simulink model "sampleModel1448_1_sub_sub_sub"  (R2023a)
settings: Solver=VariableStepAuto  StartTime=0.0  StopTime=10.0  RelTol=1e-3
libraries: hdlsllib x6, simulink x1
settings Model: Creator=user1  LastModifiedBy=user1

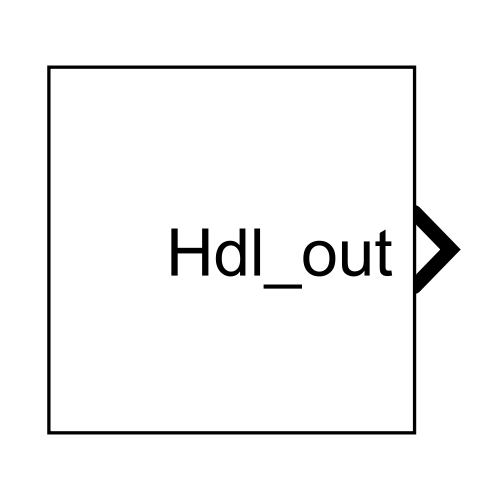
[thumbnail: Simulink's stored preview of the top-level diagram]
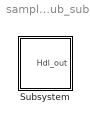
== system sampleModel1448_1_sub_sub_sub ==
  Subsystem : Subsystem

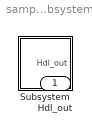
== system sampleModel1448_1_sub_sub_sub/Subsystem ==
  Subsystem : Subsystem
  Hdl_out : Outport  OutDataTypeStr=uint8

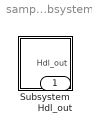
== system sampleModel1448_1_sub_sub_sub/Subsystem/Subsystem ==
  Subsystem : Subsystem
  Hdl_out : Outport  OutDataTypeStr=uint8

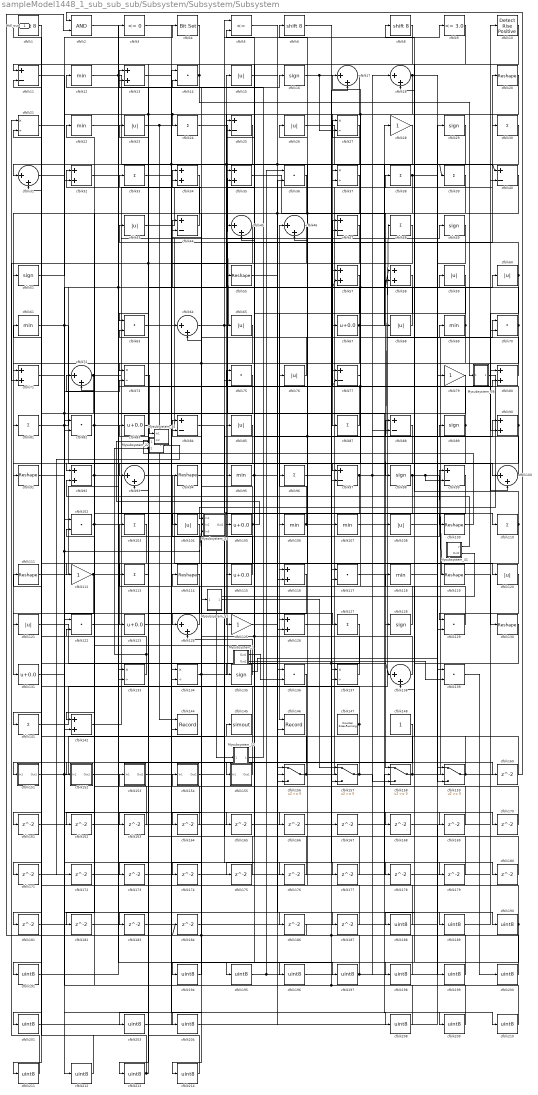
== system sampleModel1448_1_sub_sub_sub/Subsystem/Subsystem/Subsystem ==
  Mysubsystem_1 : Subsystem  TreatAsAtomicUnit=on  RTWFcnName=Mysubsystem_1
      settings: RTWFcnNameOpts=User specified  RTWFileNameOpts=Use function name
  Mysubsystem_12 : Subsystem  TreatAsAtomicUnit=on  RTWFcnName=Mysubsystem_12
      settings: RTWFcnNameOpts=User specified  RTWFileNameOpts=Use function name
  Mysubsystem_22 : Subsystem  TreatAsAtomicUnit=on  RTWFcnName=Mysubsystem_22
      settings: RTWFcnNameOpts=User specified  RTWFileNameOpts=Use function name
  Mysubsystem_23 : Subsystem  TreatAsAtomicUnit=on  RTWFcnName=Mysubsystem_23
      settings: RTWFcnNameOpts=User specified  RTWFileNameOpts=Use function name
  Mysubsystem_34 : Subsystem  TreatAsAtomicUnit=on  RTWFcnName=Mysubsystem_34
      settings: RTWFcnNameOpts=User specified  RTWFileNameOpts=Use function name
  Mysubsystem_36 : Subsystem  TreatAsAtomicUnit=on  RTWFcnName=Mysubsystem_36
      settings: RTWFcnNameOpts=User specified  RTWFileNameOpts=Use function name
  Mysubsystem_41 : Subsystem  TreatAsAtomicUnit=on  RTWFcnName=Mysubsystem_41
      settings: RTWFcnNameOpts=User specified  RTWFileNameOpts=Use function name
  Mysubsystem_51 : Subsystem  TreatAsAtomicUnit=on  RTWFcnName=Mysubsystem_51
      settings: RTWFcnNameOpts=User specified  RTWFileNameOpts=Use function name
  cfblk1 : ArithShift  BitShiftNumber=8
  cfblk10 : hdlsllib/Logic and Bit Operations/Detect Rise Positive  vinit=0  OutDataTypeStr=uint8
  cfblk{17..18,31,45..46,64,72,93,100,124,138} (11 alike) : Sum  Inputs=|++  OutDataTypeStr=uint8
  cfblk{14,36,63,70,75,82,102,117,122,129,136,139} (12 alike) : DotProduct  OutDataTypeStr=uint8
  cfblk{24,30,33,38..39,48,81,87,96,103,110,113,127,141} (14 alike) : Sum  Inputs=+  OutDataTypeStr=uint8
  cfblk{15,23,26,43,59..60,65,68,76,85,104,108,120..121} (14 alike) : Abs  OutDataTypeStr=uint8  SaturateOnIntegerOverflow=off
  cfblk{67,83,105,115,123,131} (6 alike) : Bias  Bias=0.0  SaturateOnIntegerOverflow=off
  cfblk{12,22,61,69,95,106..107,118} (8 alike) : MinMax  OutDataTypeStr=uint8
  cfblk{20,55,91,94,109,111,114,119,130} (9 alike) : Reshape
  cfblk{11,25,40,44,47,77,84,88,97,99} (10 alike) : Sum  Inputs=+-  OutDataTypeStr=uint8
  cfblk{28,79,112,125} (4 alike) : Gain  OutDataTypeStr=uint8
  cfblk{13,32,34..35,57..58,71,80,90,92,116,126,142} (13 alike) : Sum  OutDataTypeStr=uint8
  cfblk{16,29,49,51,89,98,128,135} (8 alike) : Signum
  cfblk{21,27,37,73,133..134,137} (7 alike) : Product  Inputs=*/  OutDataTypeStr=uint8  RndMeth=Zero  SaturateOnIntegerOverflow=on
  cfblk144 : Record  FileSettingsInternal="{\"entries\":[{\"content\":{\"excelSettings\":{\"content\":{},\"type\":\"Streamout.ExcelSettings\"}},\"type\":\"Streamout.FileSettingStorage\",\"uuid\":\"\"}],\"packageUris\":[\"http:\\/\\/schema.mathworks.com\\/mf0\\/streamout_blocks\\/R2020a\"],\"version\":\"1.0\"}"  Layout=[1 1]  SignalsInternal="{\"entries\":[{\"content\":{\"signals\":[{\"content\":{\"blockPath\":[],\"dimensions\":[1],\"domain\":\"\",\"lineColor\":\"#a2142f\",\"plots\":[1],\"port\":1,\"signalID\":16776,\"signalName\":\"cfblk23\"},\"type\":\"RecordBlkView.Signal\",\"uuid\":\"\"},{\"content\":{\"blockPath\":[],\"dimensions\":[1],\"domain\":\"\",\"lineColor\":\"#139fff\",\"plots\":[1],\"port\":2,\"signalID\":16779,\"signalName\":\"cfblk97\"},\"type\":\"RecordBlkView.Signal\",\"uuid\":\"\"}]},\"type\":\"RecordBlkView.InputSignals\",\"uuid\":\"\"}],\"packageUris\":[\"http:\\/\\/schema.mathworks.com\\/mf0\\/streamout_blocks\\/R2020a\"],\"version\":\"1.0\"}"  VisualizationBindings="{\"xyplotplugin\":{\"info\":[{\"series\":[{\"bindingParametersList\":[{\"parameter\":\"X-Axis\",\"signalID\":16776,\"signalName\":\"cfblk23\"},{\"parameter\":\"Y-Axis\",\"signalID\":16779,\"signalName\":\"cfblk97\"}],\"seriesID\":34221}],\"subplotID\":1}]}}"  CompatibilityTag=XY  st=-1
  cfblk145 : ToWorkspace  VariableName=simout  SaveFormat=Timeseries  SampleTime=-1
  cfblk146 : Record  FileSettingsInternal="{\"entries\":[{\"content\":{\"excelSettings\":{\"content\":{},\"type\":\"Streamout.ExcelSettings\"}},\"type\":\"Streamout.FileSettingStorage\",\"uuid\":\"\"}],\"packageUris\":[\"http:\\/\\/schema.mathworks.com\\/mf0\\/streamout_blocks\\/R2020a\"],\"version\":\"1.0\"}"  Layout=[1 1]  SignalsInternal="{\"entries\":[{\"content\":{\"signals\":[{\"content\":{\"blockPath\":[],\"dimensions\":[1],\"domain\":\"\",\"lineColor\":\"#a2142f\",\"plots\":[1],\"port\":1,\"signalID\":16784,\"signalName\":\"cfblk57\"},\"type\":\"RecordBlkView.Signal\",\"uuid\":\"\"},{\"content\":{\"blockPath\":[],\"dimensions\":[1],\"domain\":\"\",\"lineColor\":\"#139fff\",\"plots\":[1],\"port\":2,\"signalID\":16787,\"signalName\":\"cfblk29\"},\"type\":\"RecordBlkView.Signal\",\"uuid\":\"\"}]},\"type\":\"RecordBlkView.InputSignals\",\"uuid\":\"\"}],\"packageUris\":[\"http:\\/\\/schema.mathworks.com\\/mf0\\/streamout_blocks\\/R2020a\"],\"version\":\"1.0\"}"  VisualizationBindings="{\"xyplotplugin\":{\"info\":[{\"series\":[{\"bindingParametersList\":[{\"parameter\":\"X-Axis\",\"signalID\":16784,\"signalName\":\"cfblk57\"},{\"parameter\":\"Y-Axis\",\"signalID\":16787,\"signalName\":\"cfblk29\"}],\"seriesID\":57294}],\"subplotID\":1}]}}"  CompatibilityTag=XY  st=-1
  cfblk147 : hdlsllib/Sources/Counter Free-Running  NumBits=16  tsamp=-1
  cfblk148 : Constant  OutDataTypeStr=uint8  SampleTime=-1
  cfblk151 : Subsystem
      settings: LibrarySourceBlock=|
      | hdlsllib/Ports &
      | Subsystems/Subsystem
  cfblk152 : Subsystem
      settings: LibrarySourceBlock=|
      | hdlsllib/Ports &
      | Subsystems/Subsystem
  cfblk153 : Subsystem
      settings: LibrarySourceBlock=|
      | hdlsllib/Ports &
      | Subsystems/Subsystem
  cfblk154 : Subsystem
      settings: LibrarySourceBlock=|
      | hdlsllib/Ports &
      | Subsystems/Subsystem
  cfblk155 : Subsystem
      settings: LibrarySourceBlock=|
      | hdlsllib/Ports &
      | Subsystems/Subsystem
  cfblk{156..159} (4 alike) : Switch  OutDataTypeStr=uint8  SaturateOnIntegerOverflow=off  InputSameDT=off
  cfblk{160..184,186..187} (27 alike) : Delay  SampleTime=1
  cfblk{188..191,194..201,203..204,208..214} (21 alike) : DataTypeConversion  OutDataTypeStr=uint8  SaturateOnIntegerOverflow=off  RndMeth=Floor
  cfblk2 : Logic  AllPortsSameDT=off  OutDataTypeStr=boolean
  cfblk3 : hdlsllib/Logic and Bit Operations/Compare To Zero  relop=<=  OutDataTypeStr=uint8
  cfblk4 : simulink/Logic and Bit Operations/Bit Set  iBit=0
      settings: LibrarySourceBlock=|
      | hdlsllib/Logic and Bit
      | Operations/Bit Set
  cfblk5 : RelationalOperator  Operator=<=  OutDataTypeStr=boolean  InputSameDT=off
  cfblk6 : ArithShift  BitShiftNumber=8
  cfblk8 : ArithShift  BitShiftNumber=8
  cfblk9 : hdlsllib/Logic and Bit Operations/Compare To Constant  relop=<=  const=3.0  OutDataTypeStr=uint8
  Hdl_out : Outport  OutDataTypeStr=uint8
  wires:
  cfblk142/1 -> cfblk49/1
  cfblk157/1 -> cfblk158/3, cfblk155/1(In1)
  cfblk134/1 -> cfblk20/1, Mysubsystem_51/1(In1)
  cfblk156/1 -> cfblk145/1, cfblk38/1
  cfblk3/1 -> cfblk190/1
  cfblk106/1 -> cfblk109/1, cfblk46/1
  cfblk34/1 -> cfblk131/1
  cfblk93/1 -> cfblk120/1
  cfblk92/1 -> cfblk112/1, cfblk110/1
  cfblk17/1 -> cfblk87/1
  cfblk89/1 -> cfblk161/1, cfblk35/1
  cfblk25/1 -> cfblk84/2, cfblk125/1
  cfblk14/1 -> cfblk11/1, Mysubsystem_36/1(In1)
  cfblk57/1 -> cfblk146/1
  cfblk46/1 -> cfblk81/1
  cfblk5/1 -> cfblk160/1, cfblk39/1
  cfblk110/1 -> cfblk174/1, cfblk58/2
  cfblk8/1 -> cfblk93/1
  cfblk88/1 -> cfblk92/1
  cfblk85/1 -> cfblk91/1
  cfblk4/1 -> cfblk133/2
  cfblk100/1 -> cfblk45/2, cfblk6/1
  cfblk83/1 -> cfblk47/1
  cfblk108/1 -> cfblk29/1
  cfblk147/1 -> cfblk211/1, cfblk44/2
  cfblk67/1 -> cfblk181/1, cfblk44/1, cfblk28/1
  cfblk48/1 -> cfblk116/1
  cfblk90/1 -> cfblk204/1, cfblk47/2
  cfblk99/1 -> cfblk116/2
  cfblk115/1 -> cfblk94/1
  cfblk129/1 -> cfblk114/1
  cfblk141/1 -> cfblk60/1
  cfblk103/1 -> cfblk123/1
  cfblk76/1 -> cfblk12/1
  cfblk28/1 -> cfblk31/1
  cfblk82/1 -> cfblk182/1, cfblk58/1, cfblk16/1
  cfblk111/1 -> cfblk80/2
  cfblk158/1 -> cfblk31/2, cfblk70/1
  cfblk112/1 -> cfblk99/1, cfblk151/1(In1)
  cfblk87/1 -> cfblk13/1
  cfblk18/1 -> cfblk100/1, cfblk97/1, cfblk24/1, cfblk183/1, cfblk32/2
  cfblk51/1 -> cfblk4/1
  cfblk70/1 -> cfblk138/2, cfblk8/1
  cfblk138/1 -> cfblk96/1
  cfblk105/1 -> cfblk84/1, cfblk124/1
  cfblk13/1 -> cfblk64/1
  cfblk59/1 -> cfblk158/1
  cfblk122/1 -> cfblk197/1
  cfblk151/1(Out1) -> cfblk176/1, cfblk75/2
  cfblk35/1 -> cfblk128/1
  cfblk36/1 -> cfblk121/1
  cfblk29/1 -> cfblk65/1, cfblk146/2
  cfblk97/1 -> cfblk144/2, cfblk88/2, cfblk48/1
  cfblk38/1 -> cfblk71/1, cfblk159/1
  cfblk61/1 -> cfblk186/1, cfblk115/1
  cfblk128/1 -> cfblk27/1, cfblk77/2
  cfblk12/1 -> cfblk100/2, cfblk67/1
  cfblk77/1 -> cfblk57/2, cfblk17/1
  cfblk68/1 -> cfblk23/1
  cfblk137/1 -> cfblk45/1, cfblk34/1
  cfblk123/1 -> cfblk127/1
  cfblk81/1 -> cfblk73/2, cfblk15/1
  cfblk6/1 -> cfblk169/1, cfblk138/1
  cfblk21/1 -> cfblk210/1
  cfblk33/1 -> cfblk208/1
  cfblk102/1 -> cfblk168/1, cfblk22/1
  cfblk9/1 -> cfblk135/1
  cfblk139/1 -> cfblk200/1
  cfblk2/1 -> cfblk157/2
  cfblk133/1 -> cfblk111/1, Mysubsystem_22/2(In2)
  cfblk72/1 -> cfblk142/2, cfblk30/1
  cfblk39/1 -> cfblk106/1, cfblk194/1, cfblk126/2
  cfblk120/1 -> cfblk129/1
  cfblk98/1 -> cfblk99/2, cfblk119/1, cfblk152/1(In1), cfblk105/1
  cfblk117/1 -> cfblk69/1
  cfblk44/1 -> cfblk32/1
  cfblk159/1 -> cfblk118/1, cfblk2/1
  cfblk124/1 -> cfblk103/1
  cfblk20/1 -> cfblk95/1
  cfblk148/1 -> cfblk157/3
  cfblk121/1 -> cfblk156/2
  cfblk94/1 -> cfblk98/1
  cfblk95/1 -> cfblk35/2, cfblk89/1
  cfblk32/1 -> cfblk85/1
  cfblk64/1 -> cfblk9/1, cfblk108/1
  cfblk119/1 -> cfblk130/1
  cfblk118/1 -> cfblk90/1
  cfblk135/1 -> cfblk124/2
  cfblk60/1 -> cfblk43/1, cfblk90/2
  cfblk27/1 -> cfblk76/1
  cfblk113/1 -> cfblk213/1
  cfblk37/1 -> cfblk137/2
  cfblk114/1 -> cfblk134/2
  cfblk155/1(Out1) -> cfblk61/1
  cfblk24/1 -> cfblk107/1
  cfblk43/1 -> cfblk25/1
  cfblk69/1 -> cfblk18/2, cfblk164/1, cfblk163/1
  cfblk23/1 -> cfblk144/1, cfblk55/1, cfblk40/1
  cfblk30/1 -> cfblk63/1
  cfblk49/1 -> cfblk159/2
  cfblk131/1 -> cfblk59/1
  cfblk152/1(Out1) -> cfblk75/1
  cfblk1/1 -> cfblk51/1
  cfblk47/1 -> cfblk71/2, cfblk73/1
  cfblk80/1 -> cfblk5/2
  cfblk75/1 -> cfblk82/2, cfblk141/1
  cfblk40/1 -> cfblk72/2
  cfblk79/1 -> cfblk195/1
  cfblk154/1(Out1) -> cfblk88/1
  cfblk11/1 -> cfblk126/1
  cfblk22/1 -> cfblk104/1
  cfblk26/1 -> cfblk68/1
  cfblk16/1 -> cfblk179/1, cfblk27/2
  cfblk160/1 -> cfblk133/1
  cfblk161/1 -> cfblk156/1
  cfblk65/1 -> cfblk162/1
  cfblk162/1 -> cfblk37/2
  cfblk163/1 -> cfblk72/1
  cfblk164/1 -> cfblk63/2
  cfblk71/1 -> cfblk165/1
  cfblk165/1 -> cfblk77/1
  cfblk153/1(Out1) -> cfblk166/1
  cfblk166/1 -> cfblk46/2
  cfblk126/1 -> cfblk167/1
  cfblk167/1 -> cfblk40/2
  cfblk169/1 -> cfblk13/2
  cfblk96/1 -> cfblk170/1
  cfblk170/1 -> cfblk34/2
  cfblk45/1 -> cfblk171/1
  cfblk171/1 -> cfblk137/1
  cfblk172/1 -> cfblk117/2
  cfblk116/1 -> cfblk173/1
  cfblk173/1 -> cfblk158/2
  cfblk174/1 -> cfblk80/1
  cfblk58/1 -> cfblk175/1
  cfblk175/1 -> cfblk5/1
  cfblk176/1 -> cfblk64/2
  cfblk125/1 -> cfblk177/1
  cfblk177/1 -> cfblk25/2
  cfblk84/1 -> cfblk178/1
  cfblk178/1 -> cfblk70/2
  cfblk179/1 -> cfblk93/2
  cfblk31/1 -> cfblk180/1
  cfblk180/1 -> cfblk134/1
  cfblk181/1 -> cfblk129/2
  cfblk182/1 -> cfblk156/3
  cfblk183/1 -> cfblk36/2
  cfblk184/1 -> cfblk17/2
  cfblk186/1 -> cfblk2/2
  cfblk55/1 -> cfblk187/1
  cfblk187/1 -> cfblk1/1
  cfblk10/1 -> cfblk188/1
  cfblk188/1 -> cfblk26/1
  cfblk15/1 -> cfblk189/1
  cfblk189/1 -> cfblk10/1
  cfblk190/1 -> cfblk214/1, cfblk83/1
  cfblk104/1 -> cfblk191/1
  cfblk191/1 -> cfblk3/1
  cfblk195/1 -> cfblk36/1, cfblk97/2
  cfblk63/1 -> cfblk196/1
  cfblk196/1 -> cfblk79/1
  cfblk197/1 -> cfblk18/1, cfblk37/1, cfblk82/1
  cfblk130/1 -> cfblk198/1
  cfblk198/1 -> cfblk122/1
  cfblk168/1 -> cfblk199/1
  cfblk199/1 -> cfblk122/2
  cfblk200/1 -> cfblk117/1, cfblk154/1(In1), cfblk184/1
  cfblk127/1 -> cfblk201/1
  cfblk201/1 -> cfblk139/1
  cfblk136/1 -> cfblk203/1
  cfblk203/1 -> cfblk14/1
  cfblk204/1 -> cfblk136/1
  cfblk208/1 -> cfblk102/2, cfblk57/1
  cfblk107/1 -> cfblk209/1
  cfblk209/1 -> cfblk33/1
  cfblk210/1 -> cfblk102/1, Mysubsystem_23/3(In3)
  cfblk211/1 -> cfblk21/1
  cfblk91/1 -> cfblk212/1
  cfblk212/1 -> cfblk21/2
  cfblk213/1 -> cfblk153/1(In1), cfblk11/2
  cfblk214/1 -> cfblk113/1
  Mysubsystem_1/1(Out1) -> cfblk136/2
  Mysubsystem_1/2(Out2) -> cfblk139/2
  Mysubsystem_1/3(Out3) -> cfblk142/1
  Mysubsystem_1/4(Out4) -> cfblk159/3
  Mysubsystem_12/1(Out1) -> cfblk14/2
  Mysubsystem_22/1(Out1) -> cfblk172/1
  cfblk194/1 -> Mysubsystem_23/2(In2)
  Mysubsystem_23/1(Out1) -> Mysubsystem_22/1(In1)
  cfblk73/1 -> Mysubsystem_34/1(In1)
  cfblk109/1 -> Mysubsystem_34/2(In2)
  Mysubsystem_36/1(Out1) -> Mysubsystem_23/1(In1)
  Mysubsystem_41/1(y) -> cfblk92/2
  Mysubsystem_41/2(Out2) -> Mysubsystem_12/1(In1)
  Mysubsystem_51/1(Out1) -> cfblk157/1

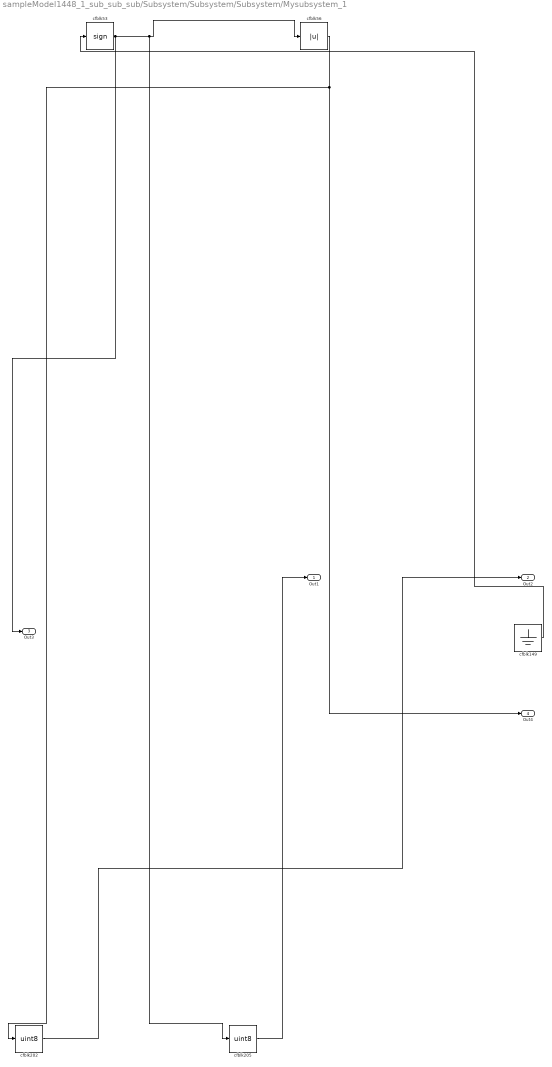
== system sampleModel1448_1_sub_sub_sub/Subsystem/Subsystem/Subsystem/Mysubsystem_1 ==
  cfblk149 : Ground
  cfblk202 : DataTypeConversion  OutDataTypeStr=uint8  SaturateOnIntegerOverflow=off  RndMeth=Floor
  cfblk205 : DataTypeConversion  OutDataTypeStr=uint8  SaturateOnIntegerOverflow=off  RndMeth=Floor
  cfblk53 : Signum
  cfblk56 : Abs  SaturateOnIntegerOverflow=off
  Out1 : Outport
  Out2 : Outport  Port=2
  Out3 : Outport  Port=3
  Out4 : Outport  Port=4
  wires:
  cfblk205/1 -> Out1/1
  cfblk202/1 -> Out2/1
  cfblk56/1 -> cfblk202/1, Out4/1
  cfblk53/1 -> cfblk205/1, cfblk56/1, Out3/1
  cfblk149/1 -> cfblk53/1

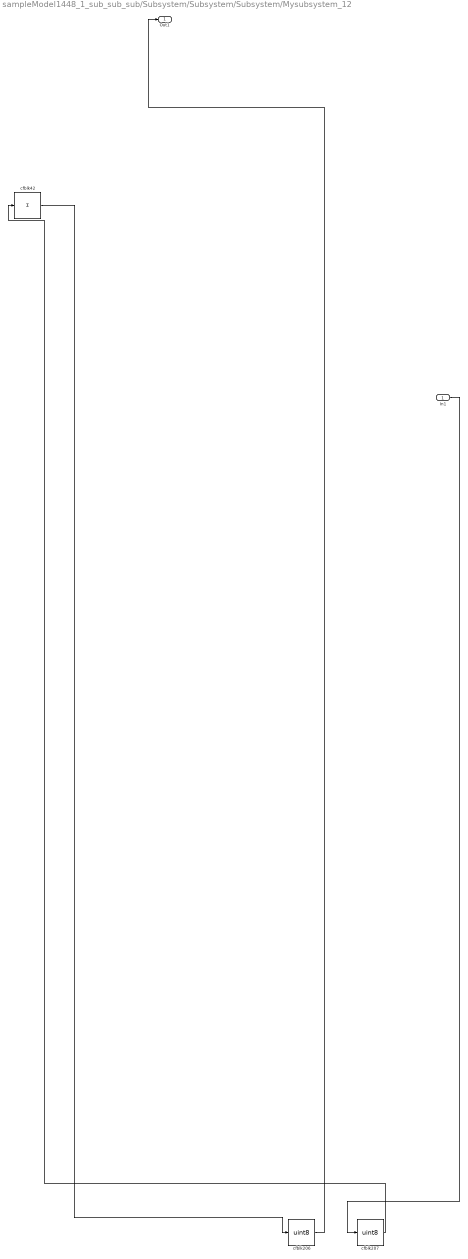
== system sampleModel1448_1_sub_sub_sub/Subsystem/Subsystem/Subsystem/Mysubsystem_12 ==
  In1 : Inport
  cfblk206 : DataTypeConversion  OutDataTypeStr=uint8  SaturateOnIntegerOverflow=off  RndMeth=Floor
  cfblk207 : DataTypeConversion  OutDataTypeStr=uint8  SaturateOnIntegerOverflow=off  RndMeth=Floor
  cfblk42 : Sum  Inputs=+
  Out1 : Outport
  wires:
  cfblk206/1 -> Out1/1
  In1/1 -> cfblk207/1
  cfblk42/1 -> cfblk206/1
  cfblk207/1 -> cfblk42/1

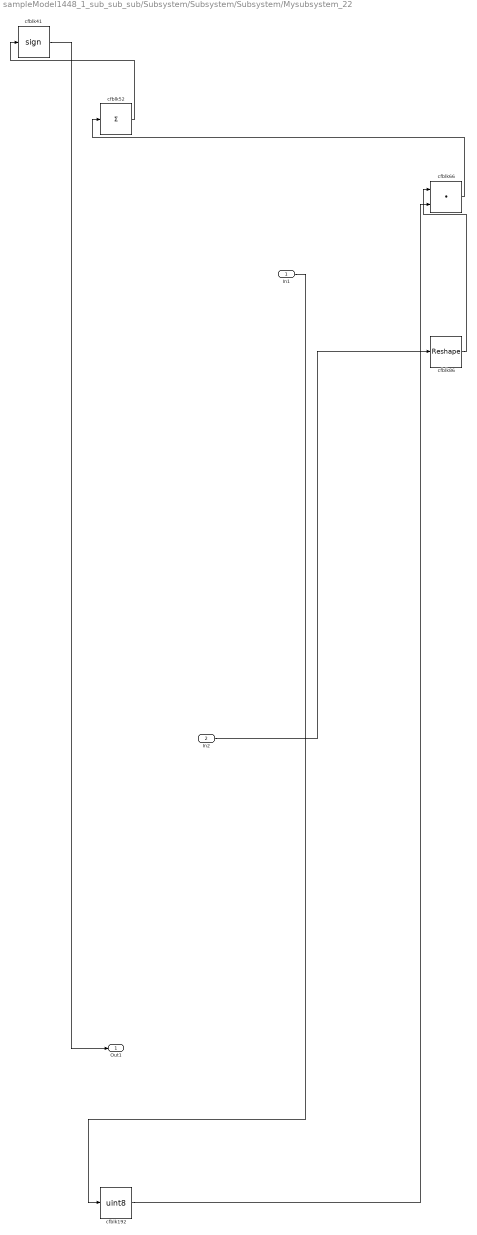
== system sampleModel1448_1_sub_sub_sub/Subsystem/Subsystem/Subsystem/Mysubsystem_22 ==
  In1 : Inport
  In2 : Inport  Port=2
  cfblk192 : DataTypeConversion  OutDataTypeStr=uint8  SaturateOnIntegerOverflow=off  RndMeth=Floor
  cfblk41 : Signum
  cfblk52 : Sum  Inputs=+
  cfblk66 : DotProduct  OutDataTypeStr=Inherit: Inherit via internal rule
  cfblk86 : Reshape
  Out1 : Outport
  wires:
  In2/1 -> cfblk86/1
  cfblk66/1 -> cfblk52/1
  cfblk192/1 -> cfblk66/2
  cfblk41/1 -> Out1/1
  In1/1 -> cfblk192/1
  cfblk52/1 -> cfblk41/1
  cfblk86/1 -> cfblk66/1

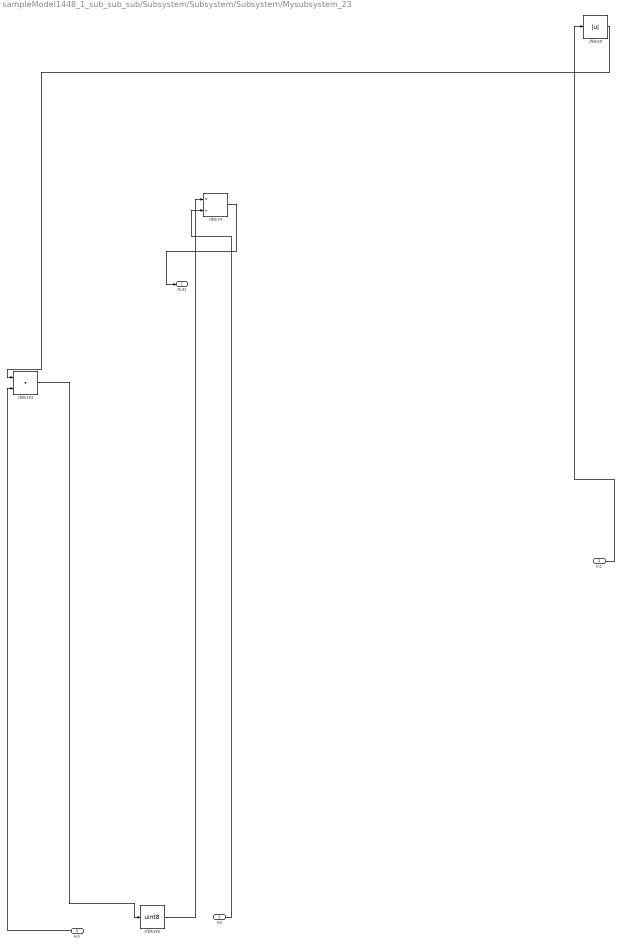
== system sampleModel1448_1_sub_sub_sub/Subsystem/Subsystem/Subsystem/Mysubsystem_23 ==
  In1 : Inport
  In2 : Inport  Port=2
  In3 : Inport  Port=3
  cfblk101 : DotProduct  OutDataTypeStr=Inherit: Inherit via internal rule
  cfblk193 : DataTypeConversion  OutDataTypeStr=uint8  SaturateOnIntegerOverflow=off  RndMeth=Floor
  cfblk50 : Abs  SaturateOnIntegerOverflow=off
  cfblk74 : Product  Inputs=*/  RndMeth=Zero  SaturateOnIntegerOverflow=on
  Out1 : Outport
  wires:
  In3/1 -> cfblk101/2
  In1/1 -> cfblk50/1
  cfblk74/1 -> Out1/1
  cfblk101/1 -> cfblk193/1
  cfblk50/1 -> cfblk101/1
  cfblk193/1 -> cfblk74/1
  In2/1 -> cfblk74/2

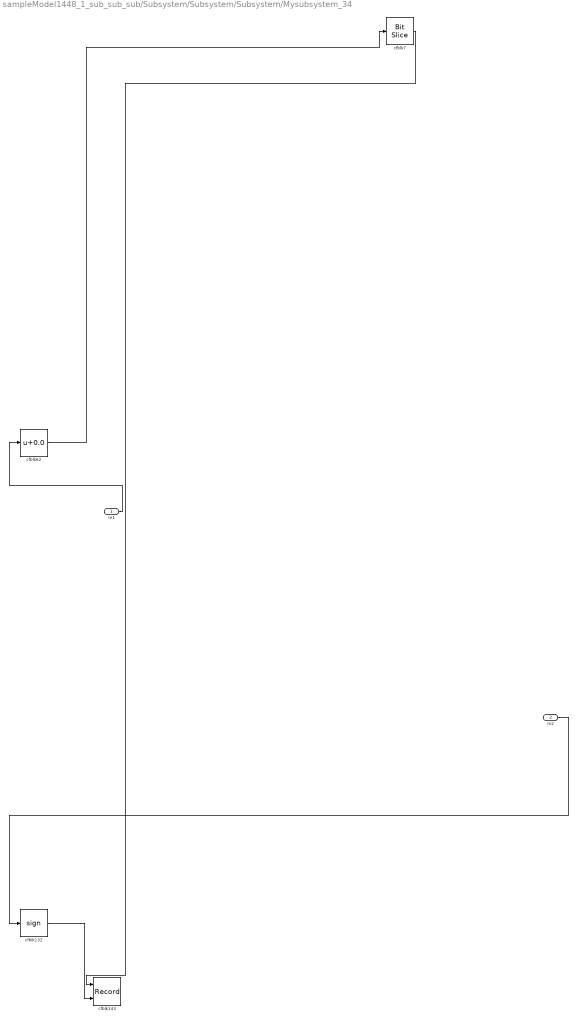
== system sampleModel1448_1_sub_sub_sub/Subsystem/Subsystem/Subsystem/Mysubsystem_34 ==
  In1 : Inport
  In2 : Inport  Port=2
  cfblk132 : Signum
  cfblk143 : Record  FileSettingsInternal="{\"entries\":[{\"content\":{\"excelSettings\":{\"content\":{},\"type\":\"Streamout.ExcelSettings\"}},\"type\":\"Streamout.FileSettingStorage\",\"uuid\":\"\"}],\"packageUris\":[\"http:\\/\\/schema.mathworks.com\\/mf0\\/streamout_blocks\\/R2020a\"],\"version\":\"1.0\"}"  Layout=[1 1]  SignalsInternal="{\"entries\":[{\"content\":{},\"type\":\"RecordBlkView.InputSignals\",\"uuid\":\"\"}],\"packageUris\":[\"http:\\/\\/schema.mathworks.com\\/mf0\\/streamout_blocks\\/R2020a\"],\"version\":\"1.0\"}"  VisualizationBindings="{\"xyplotplugin\":{\"info\":[{\"series\":[],\"subplotID\":1}]}}"  CompatibilityTag=XY  st=-1
  cfblk62 : Bias  Bias=0.0  SaturateOnIntegerOverflow=off
  cfblk7 : hdlsllib/Logic and Bit Operations/Bit Slice  lidx=7  ridx=0
  wires:
  In2/1 -> cfblk132/1
  In1/1 -> cfblk62/1
  cfblk62/1 -> cfblk7/1
  cfblk7/1 -> cfblk143/1
  cfblk132/1 -> cfblk143/2

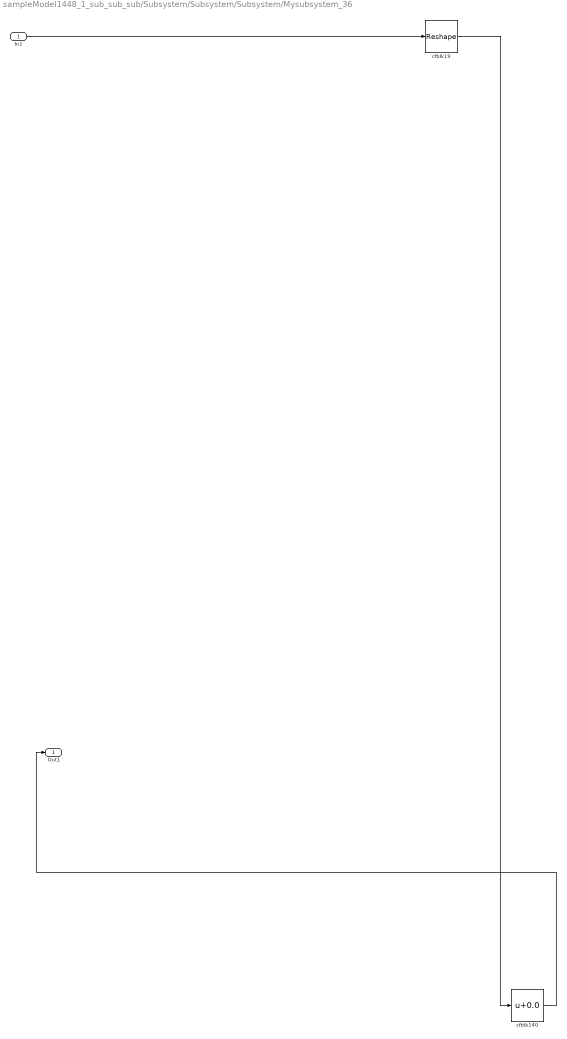
== system sampleModel1448_1_sub_sub_sub/Subsystem/Subsystem/Subsystem/Mysubsystem_36 ==
  In1 : Inport
  cfblk140 : Bias  Bias=0.0  SaturateOnIntegerOverflow=off
  cfblk19 : Reshape
  Out1 : Outport
  wires:
  cfblk140/1 -> Out1/1
  In1/1 -> cfblk19/1
  cfblk19/1 -> cfblk140/1

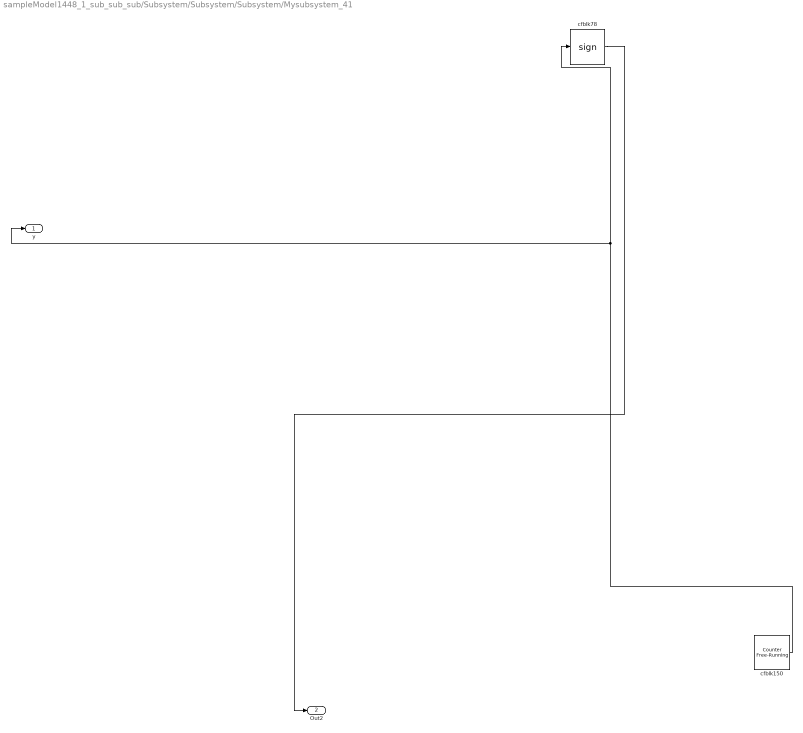
== system sampleModel1448_1_sub_sub_sub/Subsystem/Subsystem/Subsystem/Mysubsystem_41 ==
  cfblk150 : hdlsllib/Sources/Counter Free-Running  NumBits=16  tsamp=-1
  cfblk78 : Signum
  y : Outport
  Out2 : Outport  Port=2
  wires:
  cfblk78/1 -> Out2/1
  cfblk150/1 -> cfblk78/1, y/1

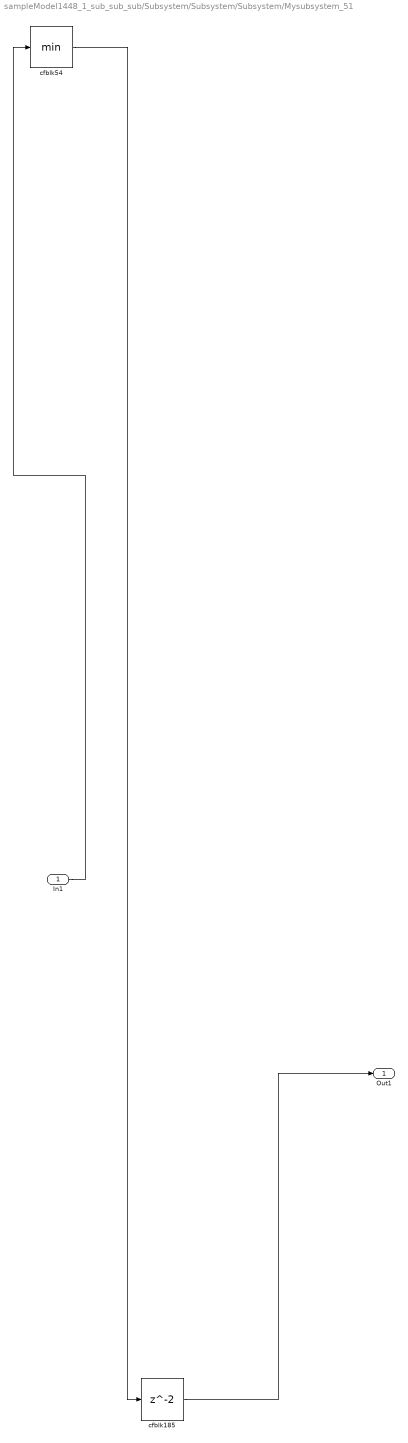
== system sampleModel1448_1_sub_sub_sub/Subsystem/Subsystem/Subsystem/Mysubsystem_51 ==
  In1 : Inport
  cfblk185 : Delay  SampleTime=1
  cfblk54 : MinMax
  Out1 : Outport
  wires:
  In1/1 -> cfblk54/1
  cfblk54/1 -> cfblk185/1
  cfblk185/1 -> Out1/1

== system sampleModel1448_1_sub_sub_sub/Subsystem/Subsystem/Subsystem/cfblk151 ==
  In1 : Inport
  Out1 : Outport
  wires:
  In1/1 -> Out1/1

== system sampleModel1448_1_sub_sub_sub/Subsystem/Subsystem/Subsystem/cfblk152 ==
  In1 : Inport
  Out1 : Outport
  wires:
  In1/1 -> Out1/1

== system sampleModel1448_1_sub_sub_sub/Subsystem/Subsystem/Subsystem/cfblk153 ==
  In1 : Inport
  Out1 : Outport
  wires:
  In1/1 -> Out1/1

== system sampleModel1448_1_sub_sub_sub/Subsystem/Subsystem/Subsystem/cfblk154 ==
  In1 : Inport
  Out1 : Outport
  wires:
  In1/1 -> Out1/1

== system sampleModel1448_1_sub_sub_sub/Subsystem/Subsystem/Subsystem/cfblk155 ==
  In1 : Inport
  Out1 : Outport
  wires:
  In1/1 -> Out1/1
